simulink model "Controller"  (R2025a)
settings: Solver=VariableStepAuto  StartTime=0.0  StopTime=10.0  RelTol=1e-3
model mask{Ts=0.01, ki=7.33, kp=9.39}
  mask prompts: Ts "Sample Time"; ki "Integral Gain"; kp "proportional Gain"
model workspace (MAT data in the model file):
  Ts = 0.01
  ki = 7.33
  kp = 9.39
undefined symbols (not defined in the file): V
settings Model: ParameterArgumentNames=Ts,ki,kp  Creator=JPIRES3  LastModifiedBy=JPIRES3
settings DataIOCC: SaveOutput=off  SaveTime=off

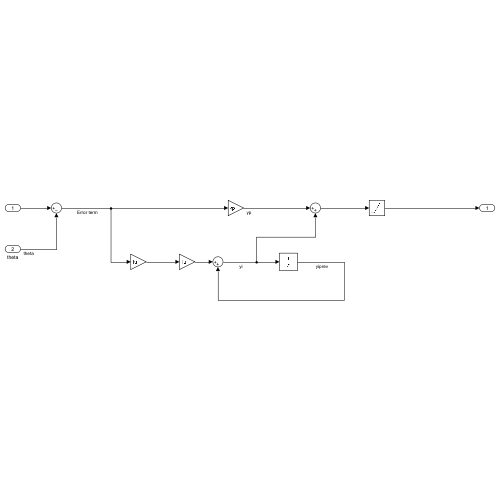
[thumbnail: Simulink's stored preview of the top-level diagram]
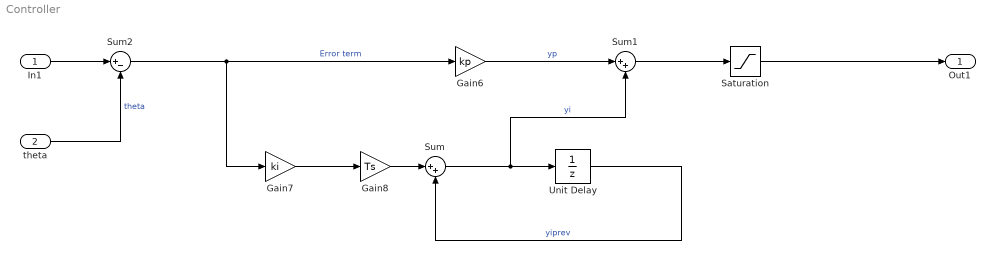
== system Controller ==
  In1 : Inport  OutDataTypeStr=double  PortDimensions=1
  theta : Inport  Port=2  OutDataTypeStr=double  PortDimensions=1  SampleTime=0
  Gain6 : Gain  Gain=kp
  Gain7 : Gain  Gain=ki
  Gain8 : Gain  Gain=Ts
  Saturation : Saturate  UpperLimit=V  LowerLimit=-V
  Sum : Sum  Inputs=|++
  Sum1 : Sum  Inputs=|++
  Sum2 : Sum  Inputs=|+-
  Unit Delay : UnitDelay  InitialCondition=1  SampleTime=Ts  HasFrameUpgradeWarning=on
  Out1 : Outport  OutDataTypeStr=double  PortDimensions=1  SampleTime=0
  wires:
  Gain8/1 -> Sum/1
  Sum/1 -> Unit Delay/1, Sum1/2  "yi"
  Sum1/1 -> Saturation/1
  Unit Delay/1 -> Sum/2  "yiprev"
  In1/1 -> Sum2/1
  Gain6/1 -> Sum1/1  "yp"
  Sum2/1 -> Gain6/1, Gain7/1  "Error term"
  Saturation/1 -> Out1/1
  Gain7/1 -> Gain8/1
  theta/1 -> Sum2/2  "theta"
